simulink model "centre_out"  (R2021a)
settings: Solver=VariableStepAuto  StartTime=0.0  StopTime=1500  RelTol=1e-3
libraries: vrlib x1
settings Model: PacingRate=0.890000  Creator=kbhar  LastModifiedBy=kbhar

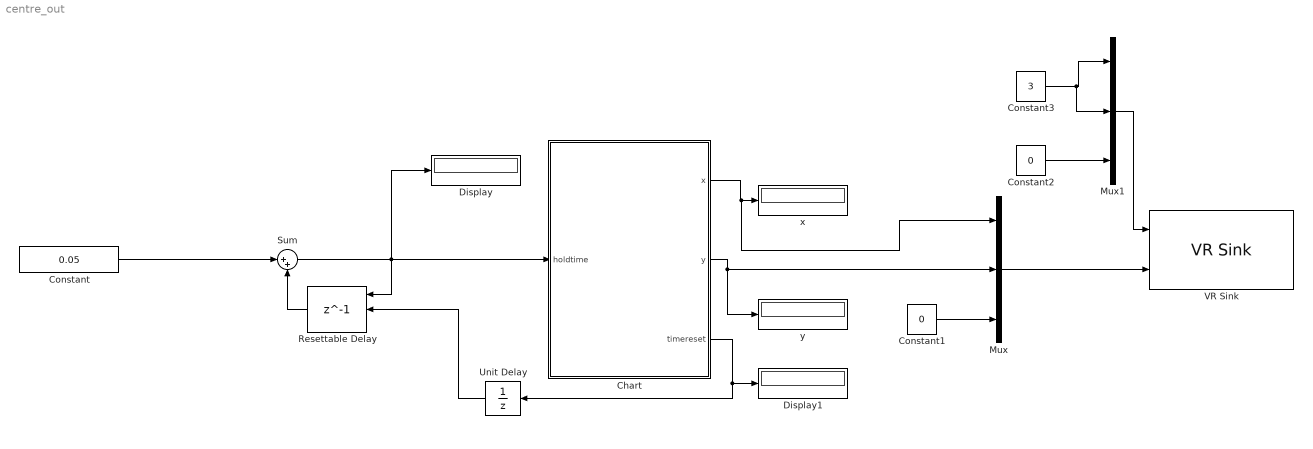
== system centre_out ==
  Chart : Stateflow chart  TreatAsAtomicUnit=on
  Constant : Constant  Value=0.05
  Constant1 : Constant  Value=0
  Constant2 : Constant  Value=0
  Constant3 : Constant  Value=3
  Display : Display
  Display1 : Display
  Mux : Mux  Inputs=3
  Mux1 : Mux  Inputs=3
  Resettable Delay : Delay  DelayLength=1  InitialConditionSource=Input port  ExternalReset=Rising
      settings: InputPortMap=u0,r5,p4
  Sum : Sum  Inputs=|++
  Unit Delay : UnitDelay  SampleTime=-1  HasFrameUpgradeWarning=on
  VR Sink : vrlib/VR Sink  InstantiateOnLoad=on  SampleTime=0.1  ViewEnable=on  RemoteChange=off  RemoteView=off  FieldsWritten=outer.translation.3.1.1.double#Cursor.translation.3.1.1.double  WorldFileName=sphere  AutoView=off  VideoDimensions=[]  AllowVariableSize=off
  x : Display
  y : Display
  wires:
  Chart/1(x) -> Mux/1, x/1
  Chart/2(y) -> y/1, Mux/2
  Sum/1 -> Chart/1(holdtime), Resettable Delay/1, Display/1
  Constant/1 -> Sum/1
  Resettable Delay/1 -> Sum/2
  Chart/3(timereset) -> Display1/1, Unit Delay/1
  Unit Delay/1 -> Resettable Delay/2
  Constant1/1 -> Mux/3
  Mux/1 -> VR Sink/2
  Constant2/1 -> Mux1/3
  Constant3/1 -> Mux1/2, Mux1/1
  Mux1/1 -> VR Sink/1

== stateflow chart centre_out/Chart ==
  state startstate
    x = 0; y = 0; timereset = 0;
  state centrestate
    x = 0; y = 0; timereset = 0;
  state resettimestate
    x = 0; y = 0; timereset = 1;
  state centrestateback
    x = 0; y = 0; timereset = 0;
  state outerstatetransition
    x = x + 0.001; y = y + 0.001; timereset = 0;
  state centrestatetransition
    x = x - 0.001; y = y - 0.001; timereset = 0;
  state outerstate
    x = 3; y = 3; timereset = 0;
  (default) -> startstate
  startstate -> centrestate
  resettimestate -> centrestate
  centrestateback -> resettimestate : [holdtime>710]
  centrestate -> outerstatetransition : [holdtime>25]
  centrestatetransition -> centrestateback : [x <= 0 && y <=0]
  outerstatetransition -> outerstate : [x >= 3 && y >= 3]
  outerstate -> centrestatetransition : [holdtime>370]
  data: x output; y output; holdtime input; timereset output
